simulink model "antiwindup_test"  (R2025b)
settings: Solver=VariableStepAuto  StartTime=0.0  StopTime=10.0  RelTol=1e-3
settings Model: Creator=lenowo twinkpad  LastModifiedBy=lenowo twinkpad

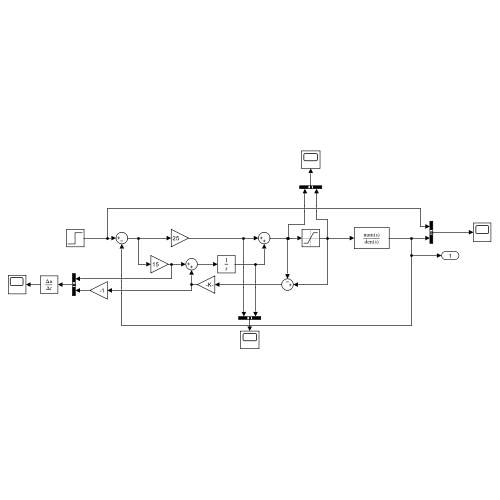
[thumbnail: Simulink's stored preview of the top-level diagram]
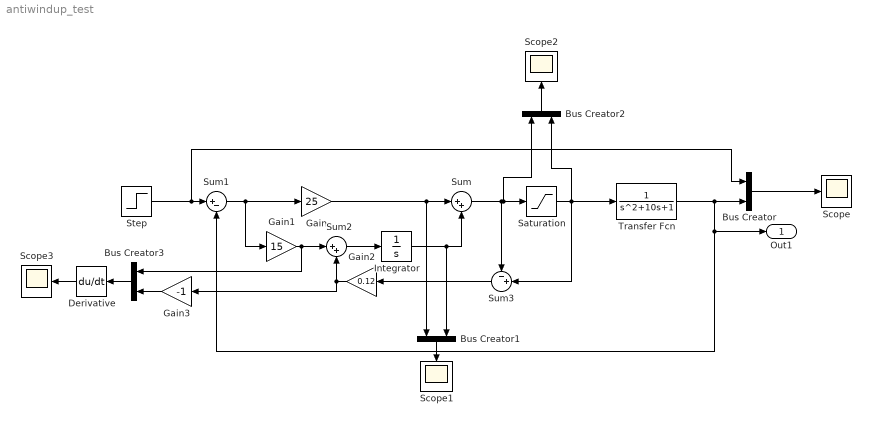
== system antiwindup_test ==
  Bus Creator{,1..3} (4 alike) : BusCreator  Inputs=2
  Derivative : Derivative
  Gain : Gain  Gain=25
  Gain1 : Gain  Gain=15
  Gain2 : Gain  Gain=0.12
  Gain3 : Gain  Gain=-1
  Integrator : Integrator
  Saturation : Saturate  UpperLimit=100  LowerLimit=-100
  Scope{,1..3} (4 alike) : Scope
      Scope settings: ActiveDisplayYMinimum=-0.15322232407907282  ActiveDisplayYMaximum=1.3790009167116557
      Scope1 settings: ActiveDisplayYMinimum=-1  ActiveDisplayYMaximum=1
      Scope2 settings: ActiveDisplayYMinimum=-1  ActiveDisplayYMaximum=1  DataLoggingVariableName=ScopeData2
      Scope3 settings: ActiveDisplayYMinimum=-5.4028100181229783  ActiveDisplayYMaximum=-1.0552955320021455  DataLoggingVariableName=ScopeData3
  Step : Step  SampleTime=0
  Sum : Sum  Inputs=|++
  Sum1 : Sum  Inputs=|+-
  Sum2 : Sum  Inputs=|++
  Sum3 : Sum  Inputs=-+|
  Transfer Fcn : TransferFcn  Denominator=[1 10 1]
  Out1 : Outport
  wires:
  Gain/1 -> Bus Creator1/1, Sum/1
  Sum/1 -> Saturation/1, Bus Creator2/1, Sum3/1
  Integrator/1 -> Sum/2, Bus Creator1/2
  Transfer Fcn/1 -> Bus Creator/2, Sum1/2, Out1/1
  Step/1 -> Bus Creator/1, Sum1/1
  Bus Creator/1 -> Scope/1
  Bus Creator1/1 -> Scope1/1
  Saturation/1 -> Sum3/2, Bus Creator2/2, Transfer Fcn/1
  Bus Creator2/1 -> Scope2/1
  Sum1/1 -> Gain1/1, Gain/1
  Sum3/1 -> Gain2/1
  Gain2/1 -> Gain3/1, Sum2/2
  Gain1/1 -> Bus Creator3/1, Sum2/1
  Sum2/1 -> Integrator/1
  Bus Creator3/1 -> Derivative/1
  Gain3/1 -> Bus Creator3/2
  Derivative/1 -> Scope3/1
